simulink model "Final_Simulation_BMWi3_Average_Model"  (R2021b)
settings: Solver=FixedStepAuto  StartTime=0.0  StopTime=10  FixedStep=Tsim  RelTol=1e-3
values from neighbouring files (symbols this model uses):
  A_front = 2.38    [parameters_BMWi3.m]
  C_drag = 0.29    [parameters_BMWi3.m]
  flux_mach = 200/(6*4800*pi/30)    (= 0.0663145596216)    [parameters_BMWi3.m]
  fr = 0.013    [parameters_BMWi3.m]
  id = I_demand .* cos(beta)    [parameters_BMWi3.m]
  Imotor_max = 400    [parameters_BMWi3.m]
  iq = I_demand .* sin(beta)    [parameters_BMWi3.m]
  J_mach = 0.0666    [parameters_BMWi3.m]
  k_gear = nmax_mach/nmax_wheel    (= 5.46098838726)    [parameters_BMWi3.m]
  Ki_id = Bw_c^2 * Ld_mach    (= 846.812057613)    [parameters_BMWi3.m]
  Ki_idc = 2*pi*BW_i*R_Lboost    (= 471.238898038)    [parameters_BMWi3.m]
  Ki_iq = Bw_c^2 * Lq_mach    (= 2368.70505626)    [parameters_BMWi3.m]
  Ki_vdc = Wn_v^2*C_boost    (= 84.3851176293)    [parameters_BMWi3.m]
  Kp_id = 2*xi_c*Bw_c*Ld_mach-R_phase_mach    [parameters_BMWi3.m]
  Kp_idc = 2*pi*BW_i*L_boost    (= 1.88495559215)    [parameters_BMWi3.m]
  Kp_iq = 2*xi_c*Bw_c*Lq_mach-R_phase_mach    [parameters_BMWi3.m]
  Kp_vdc = 2*xi*Wn_v*C_boost    [parameters_BMWi3.m]
  Ld_mach = 0.0858*1e-3    (= 8.58e-05)    [parameters_BMWi3.m]
  Lq_mach = 0.24*1e-3    (= 0.00024)    [parameters_BMWi3.m]
  mass = 1270    [parameters_BMWi3.m]
  p = 6    [parameters_BMWi3.m]
  r_wheel = (15+2*70/(100*175))*0.0254/2    (= 0.1906016)    [parameters_BMWi3.m]
  rho = 1.25    [parameters_BMWi3.m]
  T = zeros(1,length(w))    [parameters_BMWi3.m]
  T_dq = (3/2)*(p)*(flux_mach*iq+(Ld_mach-Lq_mach)*iq.*id)    [parameters_BMWi3.m]
  Tmax_mach = 250    [parameters_BMWi3.m]
  Tsim = 5e-6    (= 5e-06)    [parameters_BMWi3.m]
  Vdc = 600    [parameters_BMWi3.m]
  w = 0:1:Wmax    [parameters_BMWi3.m]
  wbase = Pmax*1e3/Tmax    (= 500)    [parameters_BMWi3.m]
undefined symbols (not defined in the file or in its folder): Ion, Lithium
libraries: nesl_utility x18, fl_lib x14, spsSecondOrderFilterLib x10, sdl_lib x8, slpidlib x7, spsMeanLib x6, simulink x4, ee_lib x4, simulink_extras x3, pid_lib x2, spsabctodq0Lib x1, drivingcycle_lib x1
(part 1 of 2)
settings Model: Creator=pawan  LastModifiedBy=pawan
settings DebuggingCC: SFMachineParentedDataDiag=warning

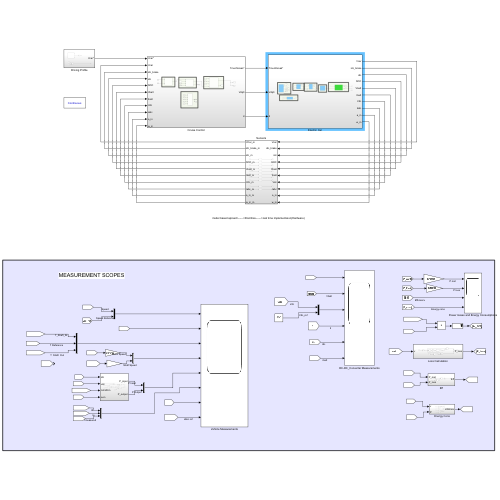
[thumbnail: Simulink's stored preview of the top-level diagram]
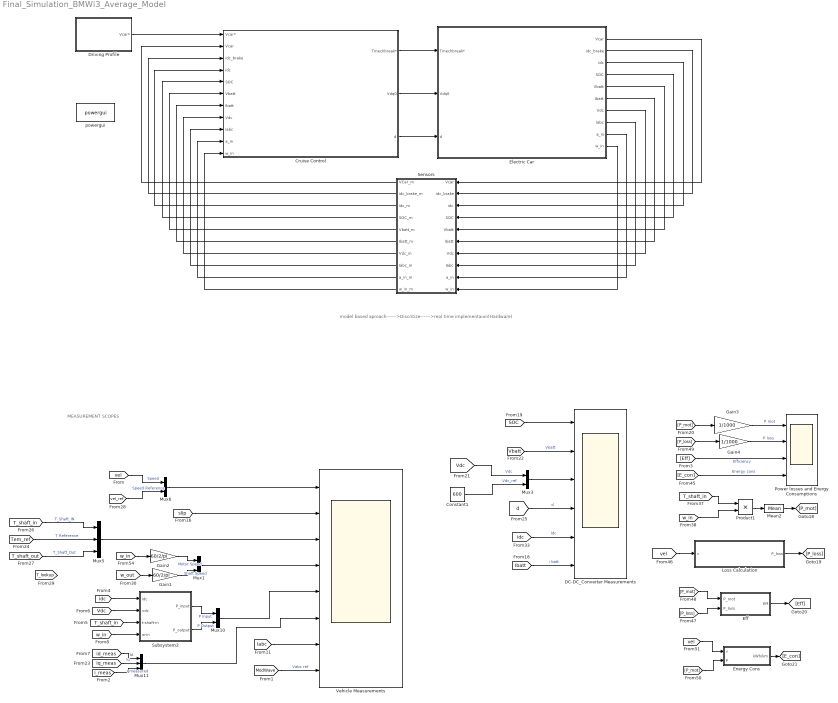
== system Final_Simulation_BMWi3_Average_Model ==
  note: MEASUREMENT SCOPES
  note: model based aproach------>Discritize------>real time implementaion(Hardware)
  Constant1 : Constant  Value=600
  Cruise Control : Subsystem
  DC-DC_Converter Measurements : Scope  NumInputPorts=6
  Driving Profile : Subsystem
  Eff : Subsystem
  Electric Car : Subsystem
  Energy Cons : Subsystem
  Gain1 : Gain  Gain=60/2/pi
  Gain2 : Gain  Gain=60/2/pi
  Gain3 : Gain  Gain=1/1000
  Gain4 : Gain  Gain=1/1000
  Loss Calculation : Subsystem
  Mean2 : spsMeanLib/Mean  Freq=50  Vinit=0  Ts=0
  Mux{1,3,6,10} (4 alike) : Mux  Inputs=2
  Mux11 : Mux  Inputs=3
  Mux5 : Mux  Inputs=3
  Power losses and Energy Consumptions : Scope  NumInputPorts=4
  Product1 : Product
  Sensors : Subsystem
  Subsystem2 : Subsystem
  Vehicle Measurements : Scope  NumInputPorts=8
  powergui : spspowerguiLib/powergui  Priority=1  SimulationMode=Continuous  SampleTime=1e-4  frequency=60  Iterations=50  frequencyindice=0  Pbase=100e6  ErrMax=1e-4  UnitsV=kV  UnitsW=MW  buscounter=0  FunctionMessages=off  echomessages=off  EnableUseOfTLC=off  CurrentSourceSwitches=off  DisableSnubberDevices=off  DisableRonSwitches=off  DisableVfSwitches=off  DisplayEquations=off  AutomaticDiscreteSolvers=off  SolverType=Tustin/Backward Euler (TBE)  Interpol=off  ExternalGateDelay=off  methode=off  Ts=100  x0status=blocks  SPID=on  SwTol=0  HookPort=off  NonlinearTolerance=1e-4  nMaxIteration=100  ContinueOnMaxIteration=off  RestoreLinks=warning  ResistiveCurrentMeasurement=off  Frange=[0:2:500]  Ylog=off  Xlog=on  ShowGrid=off  save=off  variable=ZData  structure=0  ZoomFFT=off  StartTime=0.0  cycles=1  DisplayStyle=1  fundamental=60  FreqAxis=off  MaxFrequency=1000  frequencyindicesteady=1  RmsSteady=1  display=off
  wires:
  Cruise Control/1(Tmechbreak*) -> Electric Car/1(Tmechbreak*)
  Cruise Control/2(Vdq0) -> Electric Car/2(Vdq0)
  Electric Car/1(Vcar) -> Sensors/1(Vcar)
  Sensors/1(VCar_m) -> Cruise Control/2(Vcar)
  Driving Profile/1(Vcar*) -> Cruise Control/1(Vcar*)
  Cruise Control/3(d) -> Electric Car/3(d)
  Electric Car/2(idc_brake) -> Sensors/2(idc_brake)
  Electric Car/3(idc) -> Sensors/3(idc)
  Electric Car/4(SOC) -> Sensors/4(SOC)
  Electric Car/5(Vbatt) -> Sensors/5(Vbatt)
  Electric Car/6(Ibatt) -> Sensors/6(Ibatt)
  Electric Car/7(Vdc) -> Sensors/7(Vdc)
  Electric Car/8(Iabc) -> Sensors/8(Iabc)
  Electric Car/9(a_in) -> Sensors/9(a_in)
  Electric Car/10(w_in) -> Sensors/10(w_in)
  Sensors/2(idc_brake_m) -> Cruise Control/3(idc_brake)
  Sensors/3(idc_m) -> Cruise Control/4(idc)
  Sensors/4(SOC_m) -> Cruise Control/5(SOC)
  Sensors/5(Vbatt_m) -> Cruise Control/6(Vbatt)
  Sensors/6(Ibatt_m) -> Cruise Control/7(Ibatt)
  Sensors/7(Vdc_m) -> Cruise Control/8(Vdc)
  Sensors/8(Iabc_m) -> Cruise Control/9(iabc)
  Sensors/9(a_in_m) -> Cruise Control/10(a_in)
  Sensors/10(w_in_m) -> Cruise Control/11(w_in)
  [P_mot] -> Energy Cons/2(P)
  [T_shaft_out] -> Mux5/3  "T_Shaft_Out"
  [idc] -> DC-DC_Converter Measurements/5  "Idc"
  [P_loss] -> Eff/2(P_loss)
  [w_out] -> Gain1/1
  [Eff] -> Power losses and Energy Consumptions/3  "Efficiency"
  [w_in] -> Subsystem2/4(w-in)
  Mean2/1 -> [P_mot]
  [Tem_ref] -> Mux5/2  "T Reference"
  [T_shaft_in] -> Product1/1
  [Iabc] -> Vehicle Measurements/7
  [d] -> DC-DC_Converter Measurements/4  "d"
  Energy Cons/1(kWh/km) -> [E_con]
  Product1/1 -> Mean2/1
  [vel_ref] -> Mux6/2  "Speed Reference"
  [vel] -> Mux6/1  "Speed"
  [P_mot] -> Gain3/1
  [E_con] -> Power losses and Energy Consumptions/4  "Energy cons"
  [w_in] -> Product1/2
  [P_mot] -> Eff/1(P_mot)
  [Ibatt] -> DC-DC_Converter Measurements/6  "i batt"
  Subsystem2/1(P_input) -> Mux10/1  "P Input"
  Gain3/1 -> Power losses and Energy Consumptions/1  "P mot"
  [ModWave] -> Vehicle Measurements/8  "Vabc ref"
  [Vdc] -> Mux3/1  "Vdc"
  [iq_meas] -> Mux11/2  "Iq"
  Constant1/1 -> Mux3/2  "Vdc_ref"
  Mux3/1 -> DC-DC_Converter Measurements/3
  Mux5/1 -> Vehicle Measurements/3
  Mux6/1 -> Vehicle Measurements/1
  Subsystem2/2(P_output) -> Mux10/2  "P Output"
  Gain2/1 -> Mux1/1  "Motor Speed"
  Loss Calculation/1(P_loss) -> [P_loss]
  [Vdc] -> Subsystem2/2(vdc)
  [vel] -> Loss Calculation/1(v)
  [T_shaft_in] -> Subsystem2/3(t-shaft-in)
  [idc] -> Subsystem2/1(idc)
  Eff/1(Eff) -> [Eff]
  [T_shaft_in] -> Mux5/1  "T_Shaft_IN"
  [id_meas] -> Mux11/1  "Id"
  [Vbatt] -> DC-DC_Converter Measurements/2  "Vbatt"
  [w_in] -> Gain2/1
  Mux1/1 -> Vehicle Measurements/4
  [SOC] -> DC-DC_Converter Measurements/1
  Gain1/1 -> Mux1/2  "Shaft Speed"
  Gain4/1 -> Power losses and Energy Consumptions/2  "P loss"
  [vel] -> Energy Cons/1(v)
  [P_loss] -> Gain4/1
  [slip] -> Vehicle Measurements/2
  [i_meas] -> Mux11/3  "I measured"
  Mux10/1 -> Vehicle Measurements/5
  Mux11/1 -> Vehicle Measurements/6

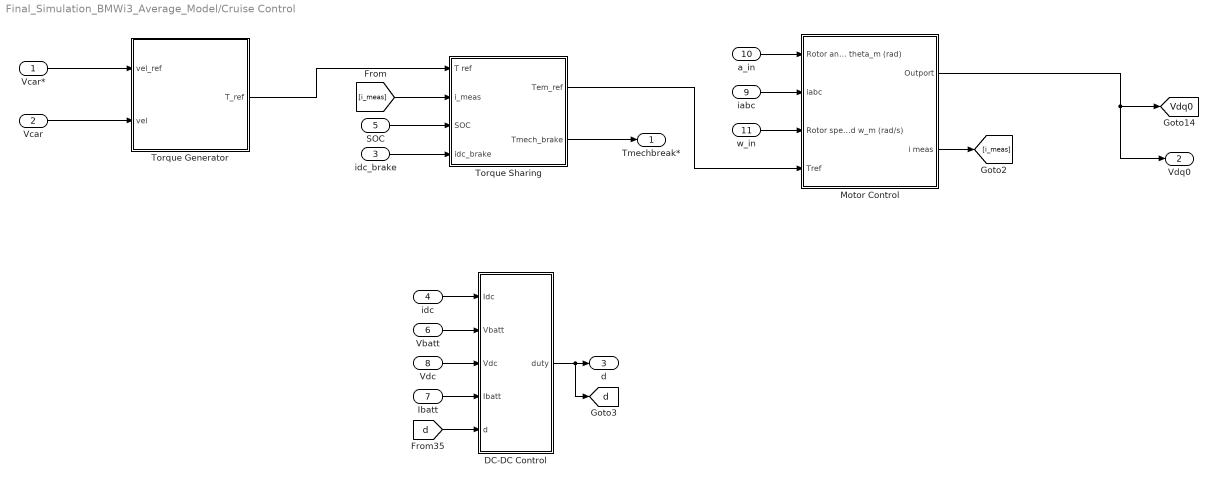
== system Final_Simulation_BMWi3_Average_Model/Cruise Control ==
  Vcar* : Inport
  Vcar : Inport  Port=2
  idc_brake : Inport  Port=3
  idc : Inport  Port=4
  SOC : Inport  Port=5
  Vbatt : Inport  Port=6
  Ibatt : Inport  Port=7
  Vdc : Inport  Port=8
  iabc : Inport  Port=9
  a_in : Inport  Port=10
  w_in : Inport  Port=11
  DC-DC Control : Subsystem
  Motor Control : Subsystem
  Torque Generator : Subsystem
  Torque Sharing : Subsystem
  Tmechbreak* : Outport
  Vdq0 : Outport  Port=2
  d : Outport  Port=3
  tag scope: Vdq0=global, d=global
  wires:
  Vcar/1 -> Torque Generator/2(vel)
  Vcar*/1 -> Torque Generator/1(vel_ref)
  idc_brake/1 -> Torque Sharing/4(idc_brake)
  Torque Sharing/2(Tmech_brake) -> Tmechbreak*/1
  SOC/1 -> Torque Sharing/3(SOC)
  [i_meas] -> Torque Sharing/2(i_meas)
  Torque Generator/1(T_ref) -> Torque Sharing/1(T ref)
  iabc/1 -> Motor Control/2(iabc)
  Torque Sharing/1(Tem_ref) -> Motor Control/4(Tref)
  w_in/1 -> Motor Control/3(Rotor speed w_m (rad/s))
  a_in/1 -> Motor Control/1(Rotor angle theta_m (rad))
  Motor Control/1(Outport) -> Vdq0/1, [Vdq0]
  [d] -> DC-DC Control/5(d)
  idc/1 -> DC-DC Control/1(Idc)
  DC-DC Control/1(duty) -> [d], d/1
  Vdc/1 -> DC-DC Control/3(Vdc)
  Vbatt/1 -> DC-DC Control/2(Vbatt)
  Ibatt/1 -> DC-DC Control/4(Ibatt)
  Motor Control/2(i meas) -> [i_meas]

== system Final_Simulation_BMWi3_Average_Model/Driving Profile ==
  note: position, speed and acceleration
  Driving Cycle : drivingcycle_lib/Driving Cycle  CycleName=WLTP class 3  CycleRepeatsForever=off
      settings: SourceProductName=Driving Cycle Blockset
  Gain : Gain  Gain=18/5
  Step1 : Step  Time=6  After=-10  SampleTime=0
  Sum8 : Sum  Inputs=|++
  Vel ref1 : Constant  Value=60
  Vcar* : Outport
  wires:
  Step1/1 -> Sum8/2
  Vel ref1/1 -> Sum8/1  "vel_ref"
  Driving Cycle/2 -> Gain/1  "m/s"
  Sum8/1 -> Vcar*/1  "Km/hr"

== system Final_Simulation_BMWi3_Average_Model/Eff ==
  P_mot : Inport
  P_loss : Inport  Port=2
  Abs : Abs
  Abs1 : Abs
  Add : Sum
  Divide : Product  Inputs=*/
  Gain : Gain  Gain=100
  Eff : Outport
  wires:
  Divide/1 -> Gain/1
  P_loss/1 -> Abs/1
  Add/1 -> Divide/2
  Abs/1 -> Add/2
  P_mot/1 -> Abs1/1
  Abs1/1 -> Add/1, Divide/1
  Gain/1 -> Eff/1

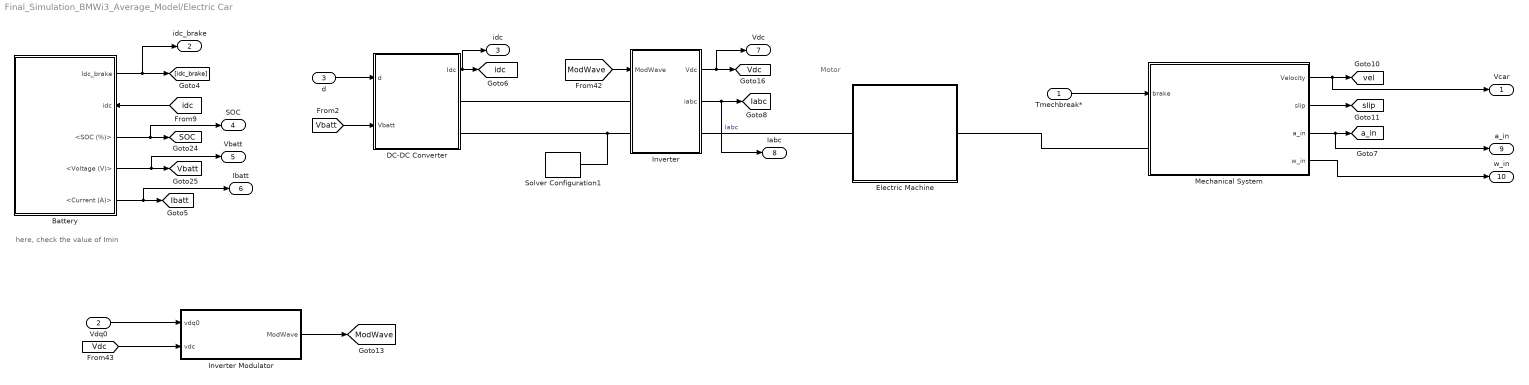
== system Final_Simulation_BMWi3_Average_Model/Electric Car ==
  note: here, check the value of Imin
  note: Motor
  Tmechbreak* : Inport
  Vdq0 : Inport  Port=2
  d : Inport  Port=3
  Battery : Subsystem
      settings: PortSchema="{\"entries\":[{\"content\":{\"sides\":[{\"content\":{\"connectorIds\":[]},\"type\":\"ConnectorPlacement.EquallySpacedRectSide\",\"uuid\":\"cc26d1cc-0fa3-4f2c-80df-1416f0a96bd3\"},{\"content\":{\"connectorIds\":[\"Out1\",\"In1\",\"Out2\",\"Out3\",\"Out4\"],\"side\":\"RIGHT\"},\"type\":\"ConnectorPlacement.EquallySpacedRectSide\",\"uuid\":\"2b739008-97af-4910-8c6c-ad69934dfbbe\"},{\"content\":{\"connectorIds\":[],\"side\":\"TOP\"},\"type\":\"ConnectorPlacement.EquallySpacedRectSide\",\"uuid\":\"d8600423-349d-4f69-80c5-5e3785c0253d\"},{\"content\":{\"connectorIds\":[],\"side\":\"HIDDEN\"},\"type\":\"ConnectorPlacement.EquallySpacedRectSide\",\"uuid\":\"c8b7a10a-4e7c-49c3-b434-bdfae66e1e22\"}]},\"type\":\"ConnectorPlacement.EquallySpacedConnector\",\"uuid\":\"b0ac5768-a943-412c-a641-9cc4a04f0544\"}],\"packageUris\":[\"http://schema.mathworks.com/mf0/Connector/R2020b\"],\"version\":\"1.0\"}"
  DC-DC Converter : Subsystem
  Electric Machine : Subsystem
  Inverter : Subsystem
  Inverter Modulator : Subsystem
  Mechanical System : Subsystem
  Solver Configuration1 : nesl_utility/Solver Configuration  PhysicalDomain=network_engine_domain  SubClassName=solver  LeftPortType=input  RightPortType=generic  Tones=[]  Harmonics=[]  SimulateNoise=off  Profile=off  UseLocalSampling=off  EnableSwitchedLinearOptims=on  FrequencyDomain=off  UseCCode=off  RelTol=0.001  AbsTol=1e-06  MinStep=1e-09  ToWorkspace=off  RevertToSquareIcSolve=off  NumHomotopyIterations=100  PhasorMode=off  PhasorModeNumHarmonics=1  DoDC=off  ResidualTolerance=1e-15  UseLocalSolver=on  LocalSolverChoice=NE_BACKWARD_EULER_ADVANCER  LocalSolverSampleTime=Tsim  DoFixedCost=on  MaxNonlinIter=3  MaxModeIter=2  ComputeImpulses=off  ImpulseIterations=2  LinearAlgebra=auto  EquationFormulation=NE_TIME_EF  DelaysMemoryBudget=1024  AutomaticFiltering=on  FilteringTimeConstant=0.001  PartitionStorageMethod=AS_NEEDED  PartitionMemoryBudget=1024  PartitionMethod=ROBUST
      settings: SourceProductBaseCode=PW,SS
  Vcar : Outport
  idc_brake : Outport  Port=2
  idc : Outport  Port=3
  SOC : Outport  Port=4
  Vbatt : Outport  Port=5
  Ibatt : Outport  Port=6
  Vdc : Outport  Port=7
  Iabc : Outport  Port=8
  a_in : Outport  Port=9
  w_in : Outport  Port=10
  tag scope: Iabc=global, Ibatt=global, ModWave=global, SOC=global, Vbatt=global, Vdc=global, a_in=global, idc=global, slip=global, vel=global
  wires:
  Vdq0/1 -> Inverter Modulator/1(vdq0)
  Inverter Modulator/1(ModWave) -> [ModWave]
  [Vdc] -> Inverter Modulator/2(vdc)
  [Vbatt] -> DC-DC Converter/2(Vbatt)
  Tmechbreak*/1 -> Mechanical System/1(brake)
  Mechanical System/4(w_in) -> w_in/1
  Mechanical System/3(a_in) -> a_in/1, [a_in]
  Inverter/2(iabc) -> Iabc/1, [Iabc]  "Iabc"
  Battery/2(<SOC (%)>) -> SOC/1, [SOC]
  Battery/4(<Current (A)>) -> Ibatt/1, [Ibatt]
  [idc] -> Battery/1(idc)
  d/1 -> DC-DC Converter/1(d)
  Inverter/1(Vdc) -> Vdc/1, [Vdc]
  [ModWave] -> Inverter/1(ModWave)
  Battery/3(<Voltage (V)>) -> Vbatt/1, [Vbatt]
  Mechanical System/2(slip) -> [slip]
  Mechanical System/1(Velocity) -> Vcar/1, [vel]
  Battery/1(Idc_brake) -> idc_brake/1, [idc_brake]
  DC-DC Converter/1(Idc) -> idc/1, [idc]
  connections:
  Inverter/LConn2 -- DC-DC Converter/RConn2 -- Solver Configuration1/RConn1
  DC-DC Converter/RConn1 -- Inverter/LConn1
  Inverter/RConn1 -- Electric Machine/LConn1
  Electric Machine/RConn1 -- Mechanical System/LConn1

== system Final_Simulation_BMWi3_Average_Model/Energy Cons ==
  v : Inport
  P : Inport  Port=2
  Clock : Clock
  Clock1 : Clock
  Distance km : Scope
  Divide : Product  Inputs=*/
  Gain1 : Gain  Gain=1/3600
  Product2 : Product
  Product3 : Product
  W to kW : Gain  Gain=1/1000
  kWh : Scope
  m/s to km/hr : Gain  Gain=18/5
  s to hr : Gain  Gain=1/3600
  kWh/km : Outport
  wires:
  Gain1/1 -> Product3/2
  s to hr/1 -> Product2/2
  m/s to km/hr/1 -> Product3/1
  Clock/1 -> s to hr/1
  Clock1/1 -> Gain1/1
  Product3/1 -> Divide/2, Distance km/1
  P/1 -> W to kW/1
  v/1 -> m/s to km/hr/1
  W to kW/1 -> Product2/1
  Product2/1 -> kWh/1, Divide/1
  Divide/1 -> kWh/km/1

== system Final_Simulation_BMWi3_Average_Model/Loss Calculation ==
  v : Inport
  Constant : Constant  Value=mass
  Gain : Gain  Gain=rho/2
  Gain1 : Gain  Gain=C_drag*A_front
  Gain2 : Gain  Gain=9.8*fr
  Gain3 : Gain  Gain=5/18
  Product : Product
  Product1 : Product
  Square : Math  Operator=square  SaturateOnIntegerOverflow=on
  Sum : Sum
  P_loss : Outport
  wires:
  Gain/1 -> Gain1/1
  Square/1 -> Gain/1
  Gain1/1 -> Product/2  "Fr"
  Product/1 -> Sum/1
  Constant/1 -> Gain2/1
  Gain2/1 -> Product1/2  "Fd"
  Product1/1 -> Sum/2
  Sum/1 -> P_loss/1
  v/1 -> Gain3/1
  Gain3/1 -> Product1/1, Product/1, Square/1

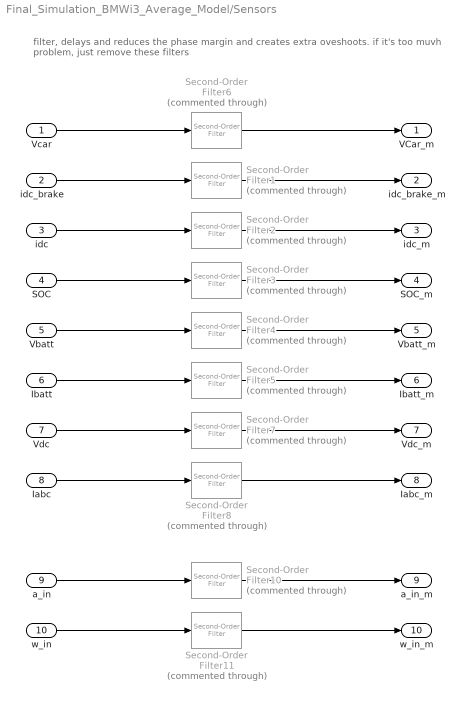
== system Final_Simulation_BMWi3_Average_Model/Sensors ==
  note: filter, delays and reduces the phase margin and creates extra oveshoots. if it's too muvh problem, just remove these filters
  Vcar : Inport
  idc_brake : Inport  Port=2
  idc : Inport  Port=3
  SOC : Inport  Port=4
  Vbatt : Inport  Port=5
  Ibatt : Inport  Port=6
  Vdc : Inport  Port=7
  Iabc : Inport  Port=8
  a_in : Inport  Port=9
  w_in : Inport  Port=10
  Second-Order Filter{1..8,10..11} (10 alike) : spsSecondOrderFilterLib/Second-Order Filter  Commented=through  FilterType=Lowpass  Fo=120  Zeta=0.707  Ts=0  Initialize=on  Vac_Init="[0,  0,  60]"  Vdc_Init=0  PlotResponse=off  FreqRange=[0, 500, 1]
      settings: SourceProductBaseCode=PS
  VCar_m : Outport
  idc_brake_m : Outport  Port=2
  idc_m : Outport  Port=3
  SOC_m : Outport  Port=4
  Vbatt_m : Outport  Port=5
  Ibatt_m : Outport  Port=6
  Vdc_m : Outport  Port=7
  Iabc_m : Outport  Port=8
  a_in_m : Outport  Port=9
  w_in_m : Outport  Port=10
  wires:
  Second-Order Filter6/1 -> VCar_m/1
  Second-Order Filter1/1 -> idc_brake_m/1
  Second-Order Filter2/1 -> idc_m/1
  Second-Order Filter4/1 -> Vbatt_m/1
  Second-Order Filter3/1 -> SOC_m/1
  Second-Order Filter5/1 -> Ibatt_m/1
  Second-Order Filter7/1 -> Vdc_m/1
  Second-Order Filter8/1 -> Iabc_m/1
  Second-Order Filter10/1 -> a_in_m/1
  Second-Order Filter11/1 -> w_in_m/1
  Vcar/1 -> Second-Order Filter6/1
  idc_brake/1 -> Second-Order Filter1/1
  idc/1 -> Second-Order Filter2/1
  SOC/1 -> Second-Order Filter3/1
  Vbatt/1 -> Second-Order Filter4/1
  Ibatt/1 -> Second-Order Filter5/1
  Vdc/1 -> Second-Order Filter7/1
  Iabc/1 -> Second-Order Filter8/1
  a_in/1 -> Second-Order Filter10/1
  w_in/1 -> Second-Order Filter11/1

== system Final_Simulation_BMWi3_Average_Model/Subsystem2 ==
  idc : Inport
  vdc : Inport  Port=2
  t-shaft-in : Inport  Port=3
  w-in : Inport  Port=4
  Constant : Constant  Value=1000
  Constant1 : Constant  Value=1000
  Divide : Product  Inputs=**
  Divide1 : Product  Inputs=**
  Divide2 : Product  Inputs=*/
  Divide3 : Product  Inputs=*/
  Mean1 : spsMeanLib/Mean  Freq=10  Vinit=0  Ts=0
  Mean2 : spsMeanLib/Mean  Freq=60  Vinit=0  Ts=0
  P_input : Outport
  P_output : Outport  Port=2
  wires:
  Divide/1 -> Mean1/1  "P_input"
  w-in/1 -> Divide1/2
  t-shaft-in/1 -> Divide1/1
  vdc/1 -> Divide/2
  Divide1/1 -> Mean2/1  "P mech output"
  idc/1 -> Divide/1
  Mean1/1 -> Divide2/1
  Divide2/1 -> P_input/1  "P_input"
  Constant/1 -> Divide2/2
  Mean2/1 -> Divide3/1
  Divide3/1 -> P_output/1  "P_output"
  Constant1/1 -> Divide3/2

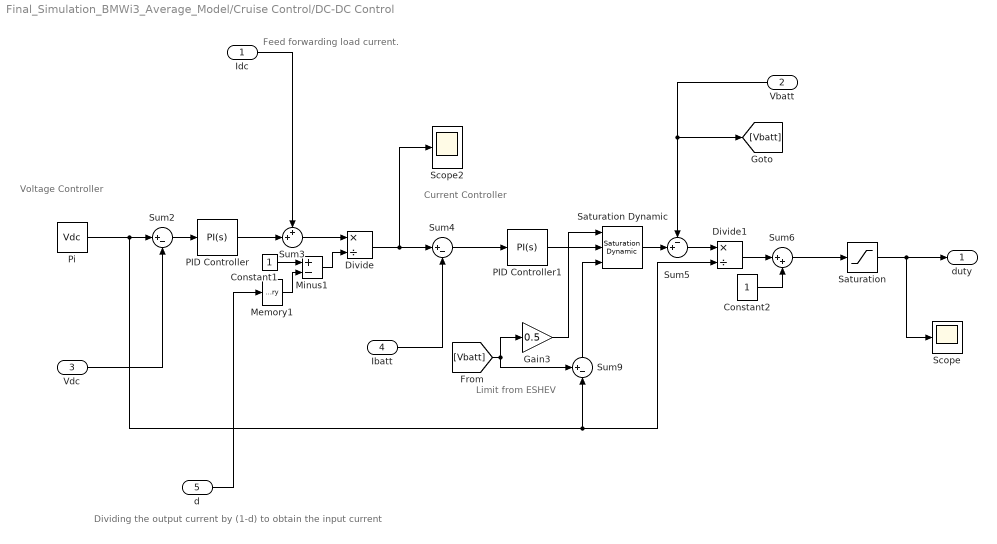
== system Final_Simulation_BMWi3_Average_Model/Cruise Control/DC-DC Control ==
  note: Limit from ESHEV
  note: Dividing the output current by (1-d) to obtain the input current
  note: Current Controller
  note: Feed forwarding load current.
  note: Voltage Controller
  Idc : Inport
  Vbatt : Inport  Port=2
  Vdc : Inport  Port=3
  Ibatt : Inport  Port=4
  d : Inport  Port=5
  Constant1 : Constant
  Constant2 : Constant
  Divide : Product  Inputs=*/
  Divide1 : Product  Inputs=*/
  Gain3 : Gain  Gain=0.5
  Memory1 : Memory
  Minus1 : Sum  Inputs=+-
  PID Controller : slpidlib/PID Controller  Controller=PI  Form=Parallel  TimeDomain=Continuous-time  UseExternalTs=off  SampleTime=-1  IntegratorMethod=Forward Euler  FilterMethod=Forward Euler  ControllerParametersSource=internal  P=Kp_vdc  I=Ki_vdc  D=0  UseFilter=on  N=100  TunerSelectOption=Transfer Function Based (PID Tuner App)  InitialConditionSource=internal  InitialConditionForIntegrator=0  InitialConditionForFilter=0  DifferentiatorICPrevScaledInput=0  ExternalReset=none  TrackingMode=off  Kt=1  LimitOutput=on  SatLimitsSource=internal  UpperSaturationLimit=400  LowerSaturationLimit=-400  LinearizeAsGain=on  AntiWindupMode=none  Kb=1  POutMin=[]  POutMax=[]  IOutMin=[]  IOutMax=[]  DOutMin=[]  DOutMax=[]  NOutMin=[]  NOutMax=[]  SumOutMin=[]  SumOutMax=[]  SaturationOutMin=[]  SaturationOutMax=[]  PParamMin=[]  PParamMax=[]  IParamMin=[]  IParamMax=[]  DParamMin=[]  DParamMax=[]  NParamMin=[]  NParamMax=[]  KbParamMin=[]  KbParamMax=[]  KtParamMin=[]  KtParamMax=[]  KbOutMin=[]  KbOutMax=[]  KtOutMin=[]  KtOutMax=[]  IntegratorOutMin=[]  IntegratorOutMax=[]  FilterOutMin=[]  FilterOutMax=[]  SumI1OutMin=[]  SumI1OutMax=[]  SumI2OutMin=[]  SumI2OutMax=[]  SumI3OutMin=[]  SumI3OutMax=[]  SumI4OutMin=[]  SumI4OutMax=[]  SumDOutMin=[]  SumDOutMax=[]  DifferentiatorOutMin=[]  DifferentiatorOutMax=[]  FilterDiffOutCoefMin=[]  FilterDiffOutCoefMax=[]  ReciprocalOutMin=[]  ReciprocalOutMax=[]  SumDenOutMin=[]  SumDenOutMax=[]  SumNumOutMin=[]  SumNumOutMax=[]  DivideOutMin=[]  DivideOutMax=[]  UdiffTsProdOutMin=[]  UdiffTsProdOutMax=[]  NTsProdOutMin=[]  NTsProdOutMax=[]  UintegralTsProdOutMin=[]  UintegralTsProdOutMax=[]  UngainTsProdOutMin=[]  UngainTsProdOutMax=[]  IntegratorContinuousStateAttributes=''  IntegratorStateMustResolveToSignalObject=off  IntegratorRTWStateStorageClass=Auto  FilterContinuousStateAttributes=''  FilterStateMustResolveToSignalObject=off  FilterRTWStateStorageClass=Auto  ParallelPVariant=InternalParameters  IdealPVariant=Disabled  IVariant=InternalParameters  DVariant=Disabled  IntegratorVariant=Continuous  SatVariant=Enabled  AWVariant=Passthrough  PCopyVariant=Disabled  TRVariant=Disabled  FdbkBlocksVariant=Forward  IdealPFdbkVariant=Disabled  SatFdbkVariant=Disabled  DerivativeFilterVariant=Disabled  NVariant=Disabled  NCopyVariant=Disabled_SignalSpec  FilterICVariant=Disabled  IntegratorICVariant=InternalICs  ExternalResetVariant=Disabled  TRSumVariant=Passthrough  SumFdbkVariant=Disabled  SumVariant=Sum_PI  TsampFilterVariant=InternalTs  TsampNgainVariant=Passthrough  TsampIntegralVariant=Passthrough  ExternalSaturationOutDataTypeStr=Inherit: Same as second input
  PID Controller1 : slpidlib/PID Controller  Controller=PI  Form=Parallel  TimeDomain=Continuous-time  UseExternalTs=off  SampleTime=-1  IntegratorMethod=Forward Euler  FilterMethod=Forward Euler  ControllerParametersSource=internal  P=Kp_idc  I=Ki_idc  D=0  UseFilter=on  N=100  TunerSelectOption=Transfer Function Based (PID Tuner App)  InitialConditionSource=internal  InitialConditionForIntegrator=0  InitialConditionForFilter=0  DifferentiatorICPrevScaledInput=0  ExternalReset=none  TrackingMode=off  Kt=1  LimitOutput=off  SatLimitsSource=internal  UpperSaturationLimit=360  LowerSaturationLimit=-360  LinearizeAsGain=on  AntiWindupMode=none  Kb=1  POutMin=[]  POutMax=[]  IOutMin=[]  IOutMax=[]  DOutMin=[]  DOutMax=[]  NOutMin=[]  NOutMax=[]  SumOutMin=[]  SumOutMax=[]  SaturationOutMin=[]  SaturationOutMax=[]  PParamMin=[]  PParamMax=[]  IParamMin=[]  IParamMax=[]  DParamMin=[]  DParamMax=[]  NParamMin=[]  NParamMax=[]  KbParamMin=[]  KbParamMax=[]  KtParamMin=[]  KtParamMax=[]  KbOutMin=[]  KbOutMax=[]  KtOutMin=[]  KtOutMax=[]  IntegratorOutMin=[]  IntegratorOutMax=[]  FilterOutMin=[]  FilterOutMax=[]  SumI1OutMin=[]  SumI1OutMax=[]  SumI2OutMin=[]  SumI2OutMax=[]  SumI3OutMin=[]  SumI3OutMax=[]  SumI4OutMin=[]  SumI4OutMax=[]  SumDOutMin=[]  SumDOutMax=[]  DifferentiatorOutMin=[]  DifferentiatorOutMax=[]  FilterDiffOutCoefMin=[]  FilterDiffOutCoefMax=[]  ReciprocalOutMin=[]  ReciprocalOutMax=[]  SumDenOutMin=[]  SumDenOutMax=[]  SumNumOutMin=[]  SumNumOutMax=[]  DivideOutMin=[]  DivideOutMax=[]  UdiffTsProdOutMin=[]  UdiffTsProdOutMax=[]  NTsProdOutMin=[]  NTsProdOutMax=[]  UintegralTsProdOutMin=[]  UintegralTsProdOutMax=[]  UngainTsProdOutMin=[]  UngainTsProdOutMax=[]  IntegratorContinuousStateAttributes=''  IntegratorStateMustResolveToSignalObject=off  IntegratorRTWStateStorageClass=Auto  FilterContinuousStateAttributes=''  FilterStateMustResolveToSignalObject=off  FilterRTWStateStorageClass=Auto  ParallelPVariant=InternalParameters  IdealPVariant=Disabled  IVariant=InternalParameters  DVariant=Disabled  IntegratorVariant=Continuous  SatVariant=Disabled  AWVariant=Passthrough  PCopyVariant=Disabled  TRVariant=Disabled  FdbkBlocksVariant=Forward  IdealPFdbkVariant=Disabled  SatFdbkVariant=Disabled  DerivativeFilterVariant=Disabled  NVariant=Disabled  NCopyVariant=Disabled_SignalSpec  FilterICVariant=Disabled  IntegratorICVariant=InternalICs  ExternalResetVariant=Disabled  TRSumVariant=Passthrough  SumFdbkVariant=Disabled  SumVariant=Sum_PI  TsampFilterVariant=InternalTs  TsampNgainVariant=Passthrough  TsampIntegralVariant=Passthrough  ExternalSaturationOutDataTypeStr=Inherit: Same as second input
  Pi : Constant  Value=Vdc  OutDataTypeStr=Inherit: Inherit via back propagation
  Saturation : Saturate  UpperLimit=1  LowerLimit=0
  Saturation Dynamic : simulink/Discontinuities/Saturation Dynamic  OutMin=[]  OutMax=[]  OutDataTypeStr=Inherit: Same as second input  OutDataType=fixdt(1, 16)  OutScaling=2^-10  DoSatur=off
  Scope : Scope
  Scope2 : Scope
  Sum2 : Sum  Inputs=|+-
  Sum3 : Sum  Inputs=++|
  Sum4 : Sum  Inputs=|+-
  Sum5 : Sum  Inputs=-+|
  Sum6 : Sum  Inputs=|++
  Sum9 : Sum  Inputs=+-|
  duty : Outport
  wires:
  Pi/1 -> Sum9/2, Divide1/2, Sum2/1
  Sum6/1 -> Saturation/1
  Divide/1 -> Scope2/1, Sum4/1
  PID Controller/1 -> Sum3/2
  Sum3/1 -> Divide/1
  Saturation Dynamic/1 -> Sum5/2
  Constant2/1 -> Sum6/2
  Vbatt/1 -> [Vbatt], Sum5/1
  PID Controller1/1 -> Saturation Dynamic/2
  Divide1/1 -> Sum6/1
  Sum9/1 -> Saturation Dynamic/3
  Ibatt/1 -> Sum4/2
  Gain3/1 -> Saturation Dynamic/1
  Sum2/1 -> PID Controller/1
  Minus1/1 -> Divide/2
  Saturation/1 -> Scope/1, duty/1
  Sum4/1 -> PID Controller1/1
  Constant1/1 -> Minus1/1
  Memory1/1 -> Minus1/2
  Sum5/1 -> Divide1/1
  Idc/1 -> Sum3/1
  Vdc/1 -> Sum2/2
  d/1 -> Memory1/1
  [Vbatt] -> Gain3/1, Sum9/1

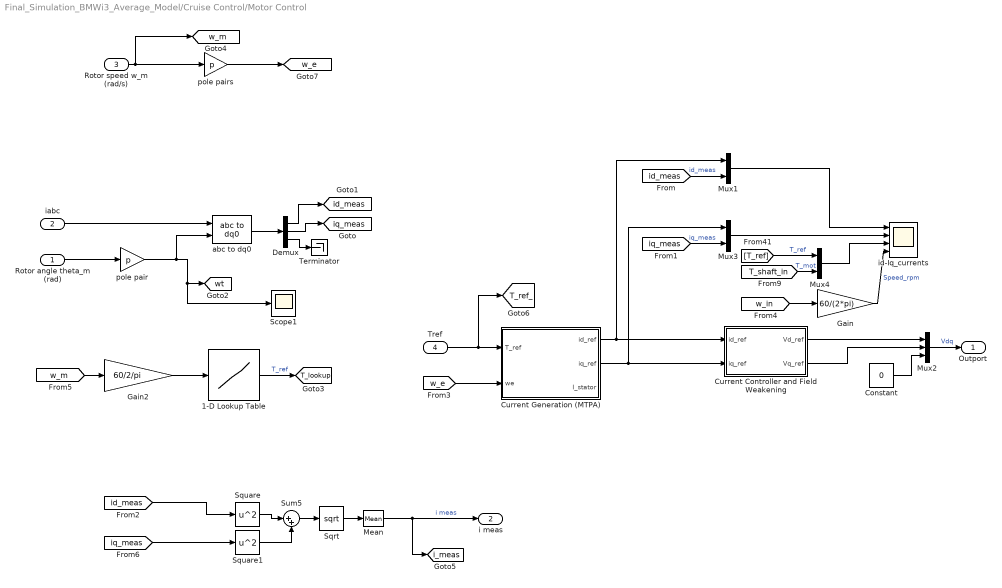
== system Final_Simulation_BMWi3_Average_Model/Cruise Control/Motor Control ==
  Rotor angle theta_m (rad) : Inport
  iabc : Inport  Port=2
  Rotor speed w_m (rad/s) : Inport  Port=3
  Tref : Inport  Port=4
  1-D Lookup Table : Lookup_n-D  NumberOfTableDimensions=1  BreakpointsForDimension1=w  Table=T  InternalRulePriority=Speed  RndMeth=Simplest  InputSameDT=on
  Constant : Constant  Value=0
  Current Controller and Field Weakening : Subsystem
  Current Generation (MTPA) : Subsystem
  Demux : Demux  Outputs=3
  Gain : Gain  Gain=60/(2*pi)
  Gain2 : Gain  Gain=60/2/pi
  Mean : spsMeanLib/Mean  Freq=60  Vinit=0  Ts=0
  Mux1 : Mux  Inputs=2
  Mux2 : Mux  Inputs=3
  Mux3 : Mux  Inputs=2
  Mux4 : Mux  Inputs=2
  Scope1 : Scope
  Sqrt : Sqrt  SaturateOnIntegerOverflow=on
  Square : Math  Operator=square  SaturateOnIntegerOverflow=on
  Square1 : Math  Operator=square  SaturateOnIntegerOverflow=on
  Sum5 : Sum  Inputs=|++
  Terminator : Terminator
  abc to dq0 : spsabctodq0Lib/abc to dq0  Alignment=90 degrees behind phase A axis
  id-Iq_currents : Scope  NumInputPorts=4
  pole pair : Gain  Gain=p
  pole pairs : Gain  Gain=p
  Outport : Outport
  i meas : Outport  Port=2
  tag scope: T_lookup=global, T_ref_=global, i_meas=global, id_meas=global, iq_meas=global, w_e=global, w_m=global, wt=global
  wires:
  Current Generation (MTPA)/1(id_ref) -> Mux1/1, Current Controller and Field Weakening/1(id_ref)
  [T_shaft_in] -> Mux4/2  "T_mot"
  pole pair/1 -> Scope1/1, [wt], abc to dq0/2
  Demux/1 -> [id_meas]
  Mux2/1 -> Outport/1  "Vdq"
  Mux1/1 -> id-Iq_currents/1
  Current Generation (MTPA)/2(iq_ref) -> Mux3/1, Current Controller and Field Weakening/2(iq_ref)
  Demux/2 -> [iq_meas]
  Gain/1 -> id-Iq_currents/4  "Speed_rpm"
  [w_e] -> Current Generation (MTPA)/2(we)
  [id_meas] -> Mux1/2  "id_meas"
  Current Controller and Field Weakening/1(Vd_ref) -> Mux2/1
  [iq_meas] -> Mux3/2  "iq_meas"
  abc to dq0/1 -> Demux/1
  Current Controller and Field Weakening/2(Vq_ref) -> Mux2/2
  Mux3/1 -> id-Iq_currents/2
  Mux4/1 -> id-Iq_currents/3
  Demux/3 -> Terminator/1
  Rotor angle theta_m (rad)/1 -> pole pair/1
  iabc/1 -> abc to dq0/1
  1-D Lookup Table/1 -> [T_lookup]  "T_ref"
  [w_in] -> Gain/1
  Gain2/1 -> 1-D Lookup Table/1
  Constant/1 -> Mux2/3
  pole pairs/1 -> [w_e]
  Rotor speed w_m (rad/s)/1 -> [w_m], pole pairs/1
  [w_m] -> Gain2/1
  [T_ref] -> Mux4/1  "T_ref"
  Tref/1 -> [T_ref_], Current Generation (MTPA)/1(T_ref)
  Square/1 -> Sum5/1
  Mean/1 -> [i_meas], i meas/1  "i meas"
  Sum5/1 -> Sqrt/1
  Square1/1 -> Sum5/2
  Sqrt/1 -> Mean/1
  [iq_meas] -> Square1/1
  [id_meas] -> Square/1

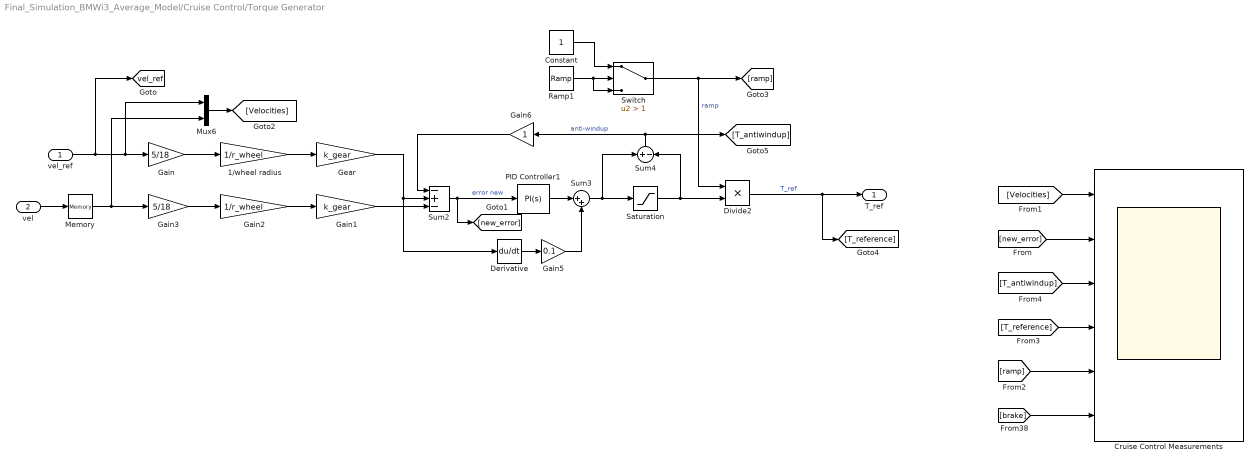
== system Final_Simulation_BMWi3_Average_Model/Cruise Control/Torque Generator ==
  vel_ref : Inport
  vel : Inport  Port=2
  1/wheel radius : Gain  Gain=1/r_wheel
  Constant : Constant
  Cruise Control Measurements : Scope  NumInputPorts=6
  Derivative : Derivative
  Divide2 : Product  Inputs=**
  Gain : Gain  Gain=5/18
  Gain1 : Gain  Gain=k_gear
  Gain2 : Gain  Gain=1/r_wheel
  Gain3 : Gain  Gain=5/18
  Gain5 : Gain  Gain=0.1
  Gain6 : Gain
  Gear : Gain  Gain=k_gear
  Memory : Memory
  Mux6 : Mux  Inputs=2
  PID Controller1 : slpidlib/PID Controller  Controller=PI  Form=Parallel  TimeDomain=Continuous-time  UseExternalTs=off  SampleTime=-1  IntegratorMethod=Forward Euler  FilterMethod=Forward Euler  ControllerParametersSource=internal  P=45  I=2  D=0  UseFilter=on  N=100  TunerSelectOption=Transfer Function Based (PID Tuner App)  InitialConditionSource=internal  InitialConditionForIntegrator=0  InitialConditionForFilter=0  DifferentiatorICPrevScaledInput=0  ExternalReset=none  TrackingMode=off  Kt=1  LimitOutput=off  SatLimitsSource=internal  UpperSaturationLimit=500  LowerSaturationLimit=-500  LinearizeAsGain=off  AntiWindupMode=clamping  Kb=1  POutMin=[]  POutMax=[]  IOutMin=[]  IOutMax=[]  DOutMin=[]  DOutMax=[]  NOutMin=[]  NOutMax=[]  SumOutMin=[]  SumOutMax=[]  SaturationOutMin=[]  SaturationOutMax=[]  PParamMin=[]  PParamMax=[]  IParamMin=[]  IParamMax=[]  DParamMin=[]  DParamMax=[]  NParamMin=[]  NParamMax=[]  KbParamMin=[]  KbParamMax=[]  KtParamMin=[]  KtParamMax=[]  KbOutMin=[]  KbOutMax=[]  KtOutMin=[]  KtOutMax=[]  IntegratorOutMin=[]  IntegratorOutMax=[]  FilterOutMin=[]  FilterOutMax=[]  SumI1OutMin=[]  SumI1OutMax=[]  SumI2OutMin=[]  SumI2OutMax=[]  SumI3OutMin=[]  SumI3OutMax=[]  SumI4OutMin=[]  SumI4OutMax=[]  SumDOutMin=[]  SumDOutMax=[]  DifferentiatorOutMin=[]  DifferentiatorOutMax=[]  FilterDiffOutCoefMin=[]  FilterDiffOutCoefMax=[]  ReciprocalOutMin=[]  ReciprocalOutMax=[]  SumDenOutMin=[]  SumDenOutMax=[]  SumNumOutMin=[]  SumNumOutMax=[]  DivideOutMin=[]  DivideOutMax=[]  UdiffTsProdOutMin=[]  UdiffTsProdOutMax=[]  NTsProdOutMin=[]  NTsProdOutMax=[]  UintegralTsProdOutMin=[]  UintegralTsProdOutMax=[]  UngainTsProdOutMin=[]  UngainTsProdOutMax=[]  IntegratorContinuousStateAttributes=''  IntegratorStateMustResolveToSignalObject=off  IntegratorRTWStateStorageClass=Auto  FilterContinuousStateAttributes=''  FilterStateMustResolveToSignalObject=off  FilterRTWStateStorageClass=Auto  ParallelPVariant=InternalParameters  IdealPVariant=Disabled  IVariant=InternalParameters  DVariant=Disabled  IntegratorVariant=Continuous  SatVariant=Disabled  AWVariant=Passthrough  PCopyVariant=Disabled  TRVariant=Disabled  FdbkBlocksVariant=Forward  IdealPFdbkVariant=Disabled  SatFdbkVariant=Disabled  DerivativeFilterVariant=Disabled  NVariant=Disabled  NCopyVariant=Disabled_SignalSpec  FilterICVariant=Disabled  IntegratorICVariant=InternalICs  ExternalResetVariant=Disabled  TRSumVariant=Passthrough  SumFdbkVariant=Disabled  SumVariant=Sum_PI  TsampFilterVariant=InternalTs  TsampNgainVariant=Passthrough  TsampIntegralVariant=Passthrough  ExternalSaturationOutDataTypeStr=Inherit: Same as second input
  Ramp1 : simulink/Sources/Ramp  slope=4  start=0  InitialOutput=0
  Saturation : Saturate  UpperLimit=Tmax_mach  LowerLimit=-Tmax_mach
  Sum2 : Sum  Inputs=-+-
  Sum3 : Sum  Inputs=|++
  Sum4 : Sum  Inputs=+|-
  Switch : Switch  Criteria=u2 > Threshold  Threshold=1
  T_ref : Outport
  tag scope: vel_ref=global
  wires:
  Constant/1 -> Switch/1
  Gain1/1 -> Sum2/3
  Sum2/1 -> [new_error], PID Controller1/1  "error new"
  Gain5/1 -> Sum3/2
  vel/1 -> Memory/1
  Sum3/1 -> Sum4/1, Saturation/1
  PID Controller1/1 -> Sum3/1
  Switch/1 -> [ramp], Divide2/1  "ramp"
  vel_ref/1 -> Gain/1, Mux6/1, [vel_ref]
  Ramp1/1 -> Switch/3, Switch/2
  Sum4/1 -> [T_antiwindup], Gain6/1  "anti-windup"
  Gain3/1 -> Gain2/1
  Divide2/1 -> [T_reference], T_ref/1  "T_ref"
  Derivative/1 -> Gain5/1
  Gear/1 -> Derivative/1, Sum2/2
  1/wheel radius/1 -> Gear/1
  Gain2/1 -> Gain1/1
  [brake] -> Cruise Control Measurements/6
  Mux6/1 -> [Velocities]
  Memory/1 -> Gain3/1, Mux6/2
  Gain/1 -> 1/wheel radius/1
  Saturation/1 -> Sum4/2, Divide2/2
  Gain6/1 -> Sum2/1
  [new_error] -> Cruise Control Measurements/2
  [Velocities] -> Cruise Control Measurements/1
  [ramp] -> Cruise Control Measurements/5
  [T_reference] -> Cruise Control Measurements/4
  [T_antiwindup] -> Cruise Control Measurements/3

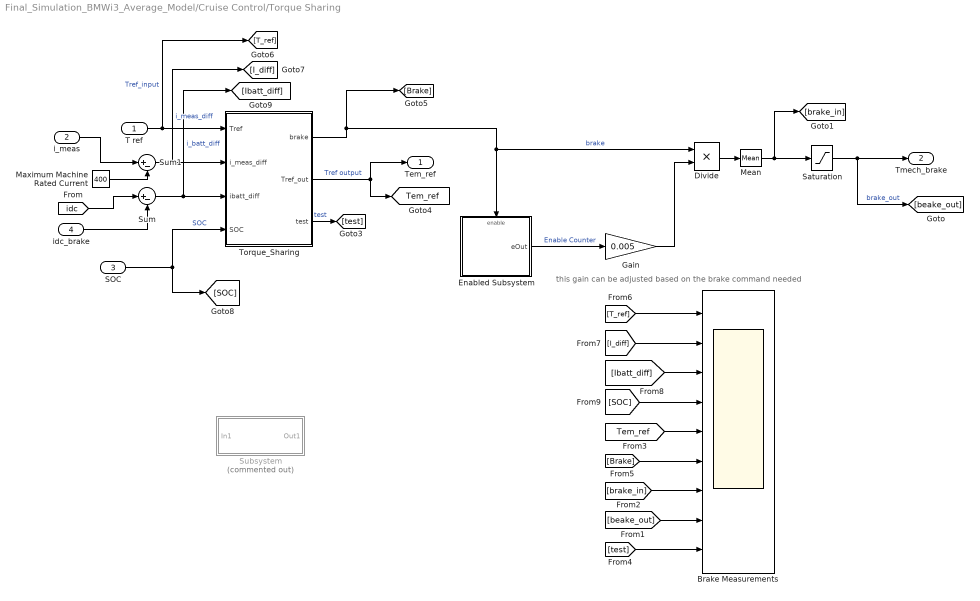
== system Final_Simulation_BMWi3_Average_Model/Cruise Control/Torque Sharing ==
  note: this gain can be adjusted based on the brake command needed
  T ref : Inport
  i_meas : Inport  Port=2
  SOC : Inport  Port=3
  idc_brake : Inport  Port=4
  Brake Measurements : Scope  NumInputPorts=9
  Divide : Product  Inputs=**
  Enabled Subsystem : Subsystem  TreatAsAtomicUnit=on
  Gain : Gain  Gain=0.005
  Maximum Machine Rated Current : Constant  Value=400
  Mean : spsMeanLib/Mean  Freq=5  Vinit=0  Ts=0
  Saturation : Saturate  LowerLimit=0
  Subsystem : Subsystem  Commented=on
  Sum : Sum  Inputs=|+-
  Sum1 : Sum  Inputs=|+-
  Torque_Sharing : MATLAB Function  TreatAsAtomicUnit=on
  Tem_ref : Outport
  Tmech_brake : Outport  Port=2
  tag scope: Tem_ref=global
  wires:
  T ref/1 -> [T_ref], Torque_Sharing/1(Tref)  "Tref_input"
  Torque_Sharing/1(brake) -> [Brake], Enabled Subsystem/Enable, Divide/1  "brake"
  Torque_Sharing/2(Tref_out) -> Tem_ref/1, [Tem_ref]  "Tref output"
  Sum1/1 -> [I_diff], Torque_Sharing/2(i_meas_diff)  "i_meas_diff"
  SOC/1 -> Torque_Sharing/4(SOC), [SOC]  "SOC"
  Sum/1 -> [Ibatt_diff], Torque_Sharing/3(ibatt_diff)  "i_batt_diff"
  [idc] -> Sum/1
  idc_brake/1 -> Sum/2
  i_meas/1 -> Sum1/1
  Maximum Machine Rated Current/1 -> Sum1/2
  Torque_Sharing/3(test) -> [test]  "test"
  Enabled Subsystem/1(eOut) -> Gain/1  "Enable Counter"
  Gain/1 -> Divide/2
  Divide/1 -> Mean/1
  Mean/1 -> [brake_in], Saturation/1
  Saturation/1 -> [beake_out], Tmech_brake/1  "brake_out"
  [beake_out] -> Brake Measurements/8
  [brake_in] -> Brake Measurements/7
  [Tem_ref] -> Brake Measurements/5
  [test] -> Brake Measurements/9
  [Brake] -> Brake Measurements/6
  [T_ref] -> Brake Measurements/1
  [I_diff] -> Brake Measurements/2
  [Ibatt_diff] -> Brake Measurements/3
  [SOC] -> Brake Measurements/4

== system Final_Simulation_BMWi3_Average_Model/Electric Car/Battery ==
  idc : Inport
  Battery : spsBatteryLib/Battery  BatType=Lithium-Ion  ShowTempParam=off  ThermalPreset=no  ShowAgeParam=off  NomV=Vn_bat  NomQ=Cn_bat  SOC=Initial_SOC  Batt_Tr=Bat_response  PresetModel=on  MaxQ=60  MinV=264.75  FullV=410.8875  Dis_rate=26.087  R=0.058833  Normal_OP=54.2609  expZone="[381.3762      2.947826]"  current=[6.5 13 32.5]  Units=Time  Tci=20  NomT=20  T2=-30  MaxQ2=4.8  FullV2=7.1  Normal_OP2=5.655  expZone2="[6.58           1]"  Rca=0.6  ti=2000  Dp=0  Neq0=0  Tsim=1e6  Ta1=25  Qeol=5.4*0.9  Reol=0.013333*1.2  Char_age=[2.3478, 3]  Dis_age=[2.3478, 10]  N1=1500  N2=10500  N3=1000  N4=1400  Ta2=45  N5=950
  Bus Selector2 : BusSelector  OutputSignals=SOC (%),Voltage (V),Current (A)
  Controlled Current Source : spsControlledCurrentSourceLib/Controlled Current Source  Initialize=on  Source_Type=AC  Amplitude=0  Phase=0  Frequency=0  Measurements=None
  Ground1 : spsGroundLib/Ground  LConnTagsString=a
  MATLAB Function : MATLAB Function  TreatAsAtomicUnit=on
  Memory : Memory
  Saturation Dynamic1 : simulink/Discontinuities/Saturation Dynamic  OutMin=[]  OutMax=[]  OutDataTypeStr=Inherit: Same as second input  OutDataType=fixdt(1, 16)  OutScaling=2^-10  DoSatur=off
  Idc_brake : Outport
  <SOC (%)> : Outport  Port=2
  <Voltage (V)> : Outport  Port=3
  <Current (A)> : Outport  Port=4
  wires:
  Bus Selector2/3 -> <Current (A)>/1  "<Current (A)>"
  Bus Selector2/1 -> <SOC (%)>/1  "<SOC (%)>"
  Saturation Dynamic1/1 -> Idc_brake/1, Controlled Current Source/1
  MATLAB Function/1(Ibmax) -> Saturation Dynamic1/1
  Battery/1 -> Bus Selector2/1
  [SOC] -> MATLAB Function/1(SOC)
  MATLAB Function/2(Ibmin) -> Saturation Dynamic1/3
  Bus Selector2/2 -> <Voltage (V)>/1  "<Voltage (V)>"
  idc/1 -> Memory/1
  Memory/1 -> Saturation Dynamic1/2
  connections:
  Ground1/LConn1 -- Battery/LConn2 -- Controlled Current Source/RConn1
  Battery/LConn1 -- Controlled Current Source/LConn1

== system Final_Simulation_BMWi3_Average_Model/Electric Car/DC-DC Converter ==
  d : Inport
  Vbatt : Inport  Port=2
  "Average-Value DC-DC Converter " : ee_lib/Semiconductors & Converters/Converters/Average-Value DC-DC Converter  control_option=ee.enum.converters.controlinput.dutycycle  converter_type=ee.enum.converters.dcdctype.boost  efficiency_option=ee.enum.converters.efficiency.constant  efficiency_fixed=97  i_vec=[0, 50, 400] A  efficiency_vec=[95, 95, 98]
      settings: SourceProductBaseCode=PS  InternalSimscapePortConfiguration="{\"Bottom\":[],\"Left\":[{\"id\":\"DutyCycle\",\"label\":\"DutyCycle\",\"type\":\"input\"},{\"id\":\"p1\",\"label\":\"1+\",\"type\":\"foundation.electrical.electrical\"},{\"id\":\"n1\",\"label\":\"1-\",\"type\":\"foundation.electrical.electrical\"}],\"Right\":[{\"id\":\"p2\",\"label\":\"2+\",\"type\":\"foundation.electrical.electrical\"},{\"id\":\"n2\",\"label\":\"2-\",\"type\":\"foundation.electrical.electrical\"}],\"Top\":[]}"
  Controlled Voltage Source : fl_lib/Electrical/Electrical Sources/Controlled Voltage Source
  Current Sensor : fl_lib/Electrical/Electrical Sensors/Current Sensor
  Mean : spsMeanLib/Mean  Freq=10  Vinit=0  Ts=0
  Memory : Memory
  PS-Simulink Converter : nesl_utility/PS-Simulink Converter  PhysicalDomain=network_engine_domain  SubClassName=ps_output  LeftPortType=input  RightPortType=output  PseudoPeriodic=off  Frequencies=[]  Unit=inherit  AffineConversion=off
      settings: SourceProductBaseCode=PW,SS
  Simulink-PS Converter : nesl_utility/Simulink-PS Converter  PhysicalDomain=network_engine_domain  SubClassName=ps_input  LeftPortType=input  RightPortType=output  PseudoPeriodic=off  Frequencies=[]  NoiseDistribution=none  NoiseParameters=[]  Unit=1  AffineConversion=off  FilteringAndDerivatives=provide  SimscapeFilterOrder=1  InputFilterTimeConstant=0.001  UdotUserProvided=0
      settings: SourceProductBaseCode=PW,SS
  Simulink-PS Converter2 : nesl_utility/Simulink-PS Converter  PhysicalDomain=network_engine_domain  SubClassName=ps_input  LeftPortType=input  RightPortType=output  PseudoPeriodic=off  Frequencies=[]  NoiseDistribution=none  NoiseParameters=[]  Unit=1  AffineConversion=off  FilteringAndDerivatives=provide  SimscapeFilterOrder=1  InputFilterTimeConstant=0.001  UdotUserProvided=0
      settings: SourceProductBaseCode=PW,SS
  + : PMIOPort  Side=Right
  - : PMIOPort  Port=2  Side=Right
  Idc : Outport
  wires:
  Memory/1 -> Simulink-PS Converter2/1
  d/1 -> Memory/1
  PS-Simulink Converter/1 -> Mean/1
  Vbatt/1 -> Simulink-PS Converter/1
  Mean/1 -> Idc/1
  connections:
  Current Sensor/RConn2 -- +/RConn1
  "Average-Value DC-DC Converter "/RConn1 -- Current Sensor/LConn1
  Controlled Voltage Source/RConn2 -- -/RConn1 -- "Average-Value DC-DC Converter "/RConn2 -- "Average-Value DC-DC Converter "/LConn3
  PS-Simulink Converter/LConn1 -- Current Sensor/RConn1
  "Average-Value DC-DC Converter "/LConn2 -- Controlled Voltage Source/LConn1
  Simulink-PS Converter2/RConn1 -- "Average-Value DC-DC Converter "/LConn1
  Simulink-PS Converter/RConn1 -- Controlled Voltage Source/RConn1

== system Final_Simulation_BMWi3_Average_Model/Electric Car/Electric Machine ==
  ERef Converter2 : fl_lib/Electrical/Electrical Elements/Electrical Reference
      settings: SourceProductName=Foundation Library
  MRRef IPMSM : fl_lib/Mechanical/Rotational Elements/Mechanical Rotational Reference
      settings: SourceProductName=Foundation Library
  PMSM1 : ee_lib/Electromechanical/Permanent Magnet/PMSM  port_option=ee.enum.threePhasePort.composite  winding_type=ee.enum.statorconnection.wye  machine_param=ee.enum.pmsm.parameterization.constant  nPolePairs=p  pmflux_param=ee.enum.pmflux.fluxlinkage  pm_flux_linkage=flux_mach Wb  torque_constant=Kt N*m/A  back_emf_constant=0.18 V/(rad/s)  stator_param=ee.enum.statorparam.LdLqL0  Ld=Ld_mach H  Lq=Lq_mach H  idVec=[-200, 0, 200] A  iqVec=[-200, 0, 200] A  LdMatrix=0.0002 * ones(3, 3) H  LqMatrix=0.0002 * ones(3, 3) H  PmMatrix=0.1 * ones(3, 3) Wb  ktMatrix=0.18 * ones(3, 3) N*m/A  keMatrix=0.18 * ones(3, 3) V/(rad/s)  L0=0.0001 H  Ls=0.0002 H  Lm=-0.00002 H  Ms=0.00002 H  Rs=R_phase_mach Ohm  zero_sequence=ee.enum.park.zerosequence.include  axes_param=ee.enum.rotorangle.qaxis  loss_param=ee.enum.ironloss.none  losses_oc=[0, 0, 0] W  losses_sc=[0, 0, 0] W  f_losses=60 Hz  Isc_losses=95 A  J=J_mach kg*m^2  lam=0 N*m/(rad/s)  i_d_specify=off  i_d_priority=None  i_d=0 A  i_d_nominal_specify=off  i_d_nominal_unit=A  i_d_nominal_value=1  i_q_specify=off  i_q_priority=None  i_q=0 A  i_q_nominal_specify=off  i_q_nominal_unit=A  i_q_nominal_value=1  torque_specify=off  torque_priority=None  torque=0 N*m  torque_nominal_specify=off  torque_nominal_unit=N*m  torque_nominal_value=1  angular_velocity_specify=off  angular_velocity_priority=High  angular_velocity=0 rpm  angular_velocity_nominal_specify=off  angular_velocity_nominal_unit=rpm  angular_velocity_nominal_value=1  angular_position_specify=off  angular_position_priority=High  angular_position=0 deg  angular_position_nominal_specify=off  angular_position_nominal_unit=deg  angular_position_nominal_value=1  alpha=3.93e-3 1/K  alpha_flux=-0.001 1/K  Tmeas=298.15 K  stator_thermal_mass=100 J/K  rotor_thermal_mass=200 J/K  Rm_percent_rotor=90  Rd_percent_rotor=30  temperatureA_specify=off  temperatureA_priority=High  temperatureA=25 degC  temperatureA_nominal_specify=off  temperatureA_nominal_unit=degC  temperatureA_nominal_value=1  temperatureB_specify=off  temperatureB_priority=High  temperatureB=25 degC  temperatureB_nominal_specify=off  temperatureB_nominal_unit=degC  temperatureB_nominal_value=1  temperatureC_specify=off  temperatureC_priority=High  temperatureC=25 degC  temperatureC_nominal_specify=off  temperatureC_nominal_unit=degC  temperatureC_nominal_value=1  temperatureR_specify=off  temperatureR_priority=High  temperatureR=25 degC  temperatureR_nominal_specify=off  temperatureR_nominal_unit=degC  temperatureR_nominal_value=1
      settings: InternalSimscapePortConfiguration="{\"Bottom\":[],\"Left\":[{\"id\":\"N\",\"label\":\"~\",\"type\":\"foundation.electrical.three_phase\"},{\"id\":\"n\",\"label\":\"n\",\"type\":\"foundation.electrical.electrical\"}],\"Right\":[{\"id\":\"R\",\"label\":\"R\",\"type\":\"foundation.mechanical.rotational.rotational\"},{\"id\":\"C\",\"label\":\"C\",\"type\":\"foundation.mechanical.rotational.rotational\"}],\"Top\":[]}"
  Vabc : PMIOPort  Side=Left
  R : PMIOPort  Port=2  Side=Right
  connections:
  PMSM1/RConn1 -- R/RConn1
  ERef Converter2/LConn1 -- PMSM1/LConn2
  PMSM1/RConn2 -- MRRef IPMSM/LConn1
  Vabc/RConn1 -- PMSM1/LConn1

== system Final_Simulation_BMWi3_Average_Model/Electric Car/Inverter ==
  note: Voltage Sensor
  ModWave : Inport
  "Average-Value Voltage Source Converter (Three-Phase) " : ee_lib/Semiconductors & Converters/Converters/Average-Value Voltage Source Converter (Three-Phase)  port_option=ee.enum.threePhasePort.composite  losses_parameterization=ee.enum.converters.losses.fixed  Pfixed=2e3 W  ks=0.01  kc1=1.7 V  kc2=0.01 Ohm  Ploss_vect=[100, 800, 1870, 3250, 4900] W  Irms_vect=[10, 100, 200, 300, 400] A  Vdc_nom=300 V  thermal_mass=30000 J/K  temperature_specify=off  temperature_priority=High  temperature=298.15 K  temperature_nominal_specify=off  temperature_nominal_unit=K  temperature_nominal_value=1
      settings: SourceProductBaseCode=PS  InternalSimscapePortConfiguration="{\"Bottom\":[],\"Left\":[{\"id\":\"ModWave\",\"label\":\"ModWave\",\"type\":\"input\"},{\"id\":\"N\",\"label\":\"~\",\"type\":\"foundation.electrical.three_phase\"}],\"Right\":[{\"id\":\"p\",\"label\":\"+\",\"type\":\"foundation.electrical.electrical\"},{\"id\":\"n\",\"label\":\"-\",\"type\":\"foundation.electrical.electrical\"}],\"Top\":[]}"
  Current Sensor : ee_lib/Sensors & Transducers/Current Sensor (Three-Phase)
      settings: SourceProductName=Electrical
  ERef Converter1 : fl_lib/Electrical/Electrical Elements/Electrical Reference
      settings: SourceProductName=Foundation Library
  Memory7 : Memory
  PS-Simulink Converter : nesl_utility/PS-Simulink Converter  PhysicalDomain=network_engine_domain  SubClassName=ps_output  LeftPortType=input  RightPortType=output  PseudoPeriodic=off  Frequencies=[]  Unit=inherit  AffineConversion=off
      settings: SourceProductBaseCode=PW,SS
  PS-Simulink Converter1 : nesl_utility/PS-Simulink Converter  PhysicalDomain=network_engine_domain  SubClassName=ps_output  LeftPortType=input  RightPortType=output  PseudoPeriodic=off  Frequencies=[]  Unit=inherit  AffineConversion=off
      settings: SourceProductBaseCode=PW,SS
  Simulink-PS Converter2 : nesl_utility/Simulink-PS Converter  PhysicalDomain=network_engine_domain  SubClassName=ps_input  LeftPortType=input  RightPortType=output  PseudoPeriodic=off  Frequencies=[]  NoiseDistribution=none  NoiseParameters=[]  Unit=1  AffineConversion=off  FilteringAndDerivatives=zero  SimscapeFilterOrder=1  InputFilterTimeConstant=0.001  UdotUserProvided=1
      settings: SourceProductName=Utilities
  Voltage Sensor : fl_lib/Electrical/Electrical Sensors/Voltage Sensor
      settings: SourceProductName=Foundation Library
  + : PMIOPort  Side=Left
  - : PMIOPort  Port=2  Side=Left
  Vabc : PMIOPort  Port=3  Side=Right
  Vdc : Outport
  iabc : Outport  Port=2
  wires:
  PS-Simulink Converter/1 -> Vdc/1
  PS-Simulink Converter1/1 -> iabc/1
  Memory7/1 -> Simulink-PS Converter2/1
  ModWave/1 -> Memory7/1
  connections:
  -/RConn1 -- ERef Converter1/LConn1 -- Voltage Sensor/RConn2 -- "Average-Value Voltage Source Converter (Three-Phase) "/RConn2
  "Average-Value Voltage Source Converter (Three-Phase) "/RConn1 -- +/RConn1 -- Voltage Sensor/LConn1
  Simulink-PS Converter2/RConn1 -- "Average-Value Voltage Source Converter (Three-Phase) "/LConn1
  Voltage Sensor/RConn1 -- PS-Simulink Converter/LConn1
  Current Sensor/RConn1 -- PS-Simulink Converter1/LConn1
  Vabc/RConn1 -- Current Sensor/RConn2
  "Average-Value Voltage Source Converter (Three-Phase) "/LConn2 -- Current Sensor/LConn1

== system Final_Simulation_BMWi3_Average_Model/Electric Car/Inverter Modulator ==
  vdq0 : Inport
  vdc : Inport  Port=2
  "PWM Generator (Three-phase, Two-level) " : eePwmGeneratorTwoLevel/PWM Generator (Three-phase, Two-level)  PWMMode=Continuous PWM (CPWM)  CPWMMode=SVM: space vector modulation  DPWMMode=60 DPWM: 60 degree discontinuous PWM  fsw=fsw_inv  Ts=Tsim
      settings: SourceProductBaseCode=PS
  Scope : Scope  NumInputPorts=3
  Scope2 : Scope
  dq0 to abc : spsdq0toabcLib/dq0 to abc  Alignment=90 degrees behind phase A axis
  ModWave : Outport
  wires:
  [Vdq] -> Scope/1
  "PWM Generator (Three-phase, Two-level) "/2 -> ModWave/1
  [wt] -> dq0 to abc/2
  "PWM Generator (Three-phase, Two-level) "/1 -> Scope2/1
  [ModWave] -> Scope/3
  dq0 to abc/1 -> "PWM Generator (Three-phase, Two-level) "/1, Scope/2  "Vabc_ref"
  vdq0/1 -> [Vdq], dq0 to abc/1
  vdc/1 -> "PWM Generator (Three-phase, Two-level) "/2
